simulink model "syntheticData"  (R2023a)
settings: Solver=FixedStepAuto  StartTime=0.0  StopTime=0.1  RelTol=1e-3
libraries: mjLib x2, visionsinks x2
settings Model: Creator=vmano  LastModifiedBy=vmano
settings OptimizationCC: ReuseModelBlockBuffer=off
settings SFSimCC: SimTargetLang=C++

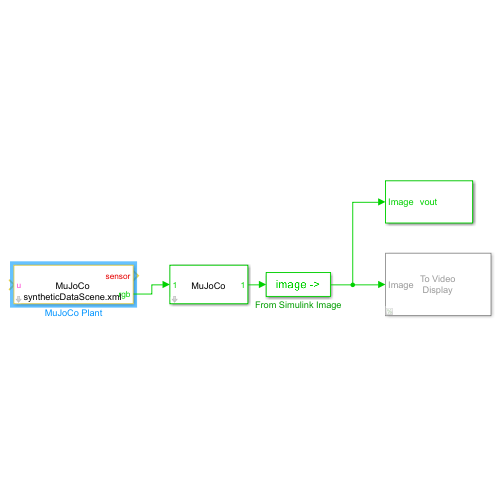
[thumbnail: Simulink's stored preview of the top-level diagram]
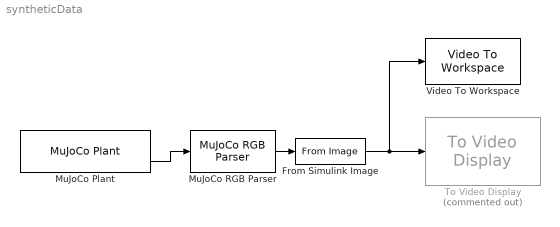
== system syntheticData ==
  From Simulink Image : FromImage
  MuJoCo Plant : mjLib/MuJoCo Plant  controlBus=[]  sensorBus=mj_bus_sensor_7979902499018342666  controlLength=[]  sensorLength=[]  rgbLength=[]  depthLength=[]  sampleTime=0.001  xmlFileRel=syntheticDataScene.xml  xmlFile=D:\manoj_stuff\mujoco-demo\examples\models\syntheticDataScene.xml  renderingType=None  vsync=off  visualFPS=60  zoomLevel=1  znear=0.03  zfar=150  cameraSampleTime=0.040  rgbOutOption=on  depthOutOption=off  controlInterfaceType=Vector
      settings: SourceProductName=MuJoCo Simulator
  MuJoCo RGB Parser : mjLib/MuJoCo RGB Parser  inputBusType=mj_bus_rgb_6905886718754851708  selectedCamera=rgbcam  imageRows=480  imageCols=640  startingIndex=1  endingIndex=921600
      settings: SourceProductName=MuJoCo Simulator
  To Video Display : visionsinks/To Video Display  Commented=on  windowSizeMode=Normal  openAtMdlStart=on  fullScreen=off  videoWindowX=2876  videoWindowY=915  saveWindowSize=off  videoWindowWidth=779  videoWindowHeight=730  inputColorFormat=RGB  inputType=Obsolete  imagePorts=One multidimensional signal  OutputDevice=On-screen video monitor  dataOrg=Column-major  isWindowOpen=off
  Video To Workspace : visionsinks/Video To Workspace  VariableName=vout  NumInputs=1  DataLimit=1  DecimationFactor=1  LogFi=off  InPortLabels=R|G|B
  wires:
  MuJoCo Plant/2 -> MuJoCo RGB Parser/1
  MuJoCo RGB Parser/1 -> From Simulink Image/1
  From Simulink Image/1 -> Video To Workspace/1, To Video Display/1
